simulink model "simulink2_dynamic_circle1"  (R2022a)
settings: Solver=FixedStepDiscrete  StartTime=0.0  StopTime=10.0  FixedStep=0.1  RelTol=1e-3
model workspace (MAT data in the model file):
  acceleration = 1
  alignment = 1
  cohesion = 1
  d_min = 0.5
  dt = 1
  eta = 1.5
  forward = 1
  k_ = 0.5
  k_tsmc = 1
  lambda_ = 2
  leader_position = [0 0 5]
  leader_velocity = [1 1 0]
  max_velocity = 5
  n_drones = 10
  neighbor_rad = 15
  radius = 10
  radius1 = 20
  ref_position = [20 20 5]
  ref_velocity = [0 0 0]
  separation = 1.5
  time_steps = 50
  u_max = 10
  velocities = [5 5 5]
  velocity = 5
settings Model: Creator=admin  LastModifiedBy=admin

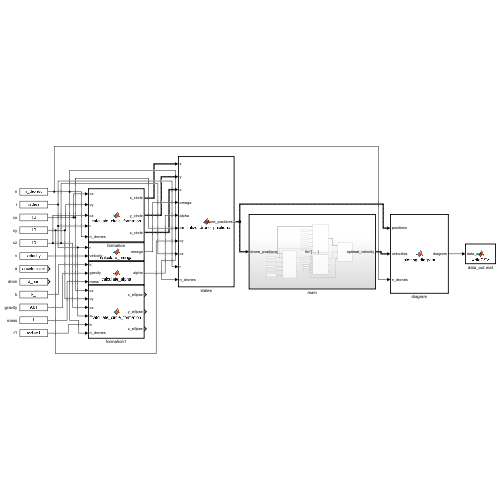
[thumbnail: Simulink's stored preview of the top-level diagram]
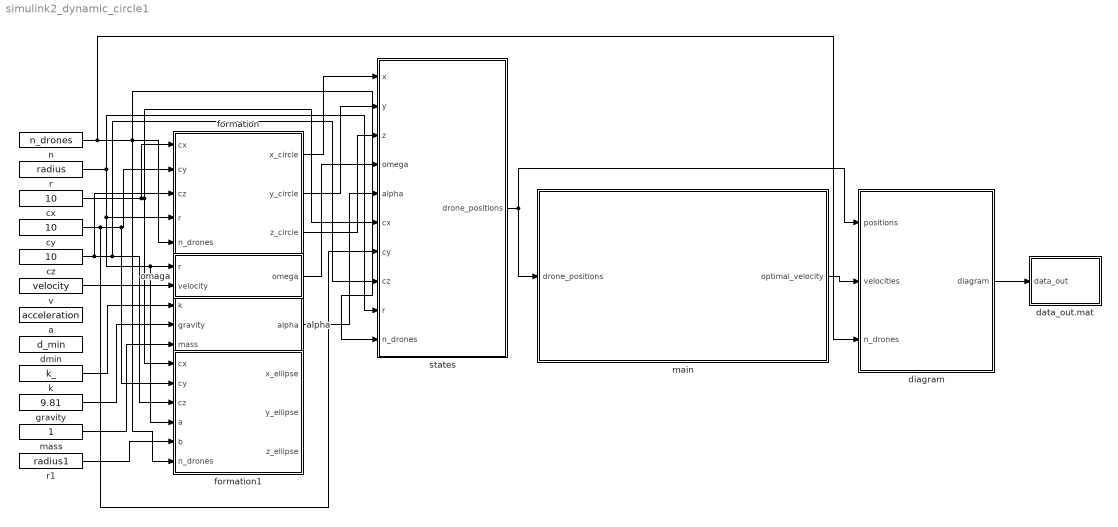
== system simulink2_dynamic_circle1 ==
  a : Constant  Value=acceleration
  alpha : MATLAB Function  TreatAsAtomicUnit=on
  cx : Constant  Value=10
  cy : Constant  Value=10
  cz : Constant  Value=10
  data_out.mat : MATLAB Function  TreatAsAtomicUnit=on
  diagram : MATLAB Function  TreatAsAtomicUnit=on
  dmin : Constant  Value=d_min
  formation : MATLAB Function  TreatAsAtomicUnit=on  SystemSampleTime=0.1
  formation1 : MATLAB Function  TreatAsAtomicUnit=on  SystemSampleTime=0.1
  gravity : Constant  Value=9.81
  k : Constant  Value=k_
  main : Subsystem  TreatAsAtomicUnit=on
  mass : Constant
  n : Constant  Value=n_drones
  omaga : MATLAB Function  TreatAsAtomicUnit=on
  r : Constant  Value=radius
  r1 : Constant  Value=radius1
  states : MATLAB Function  TreatAsAtomicUnit=on  SystemSampleTime=0.1
  v : Constant  Value=velocity
  wires:
  v/1 -> omaga/2(velocity)
  r/1 -> formation1/4(a), omaga/1(r), formation/4(r), states/9(r)
  k/1 -> alpha/1(k)
  gravity/1 -> alpha/2(gravity)
  mass/1 -> alpha/3(mass)
  cx/1 -> states/6(cx), formation1/1(cx), formation/1(cx)
  cy/1 -> states/7(cy), formation1/2(cy), formation/2(cy)
  cz/1 -> states/8(cz), formation1/3(cz), formation/3(cz)
  n/1 -> diagram/3(n_drones), states/10(n_drones), formation1/6(n_drones), formation/5(n_drones)
  r1/1 -> formation1/5(b)
  states/1(drone_positions) -> diagram/1(positions), main/1(drone_positions)
  formation/1(x_circle) -> states/1(x)
  formation/2(y_circle) -> states/2(y)
  formation/3(z_circle) -> states/3(z)
  omaga/1(omega) -> states/4(omega)
  alpha/1(alpha) -> states/5(alpha)
  main/1(optimal_velocity) -> diagram/2(velocities)
  diagram/1(diagram) -> data_out.mat/1(data_out)

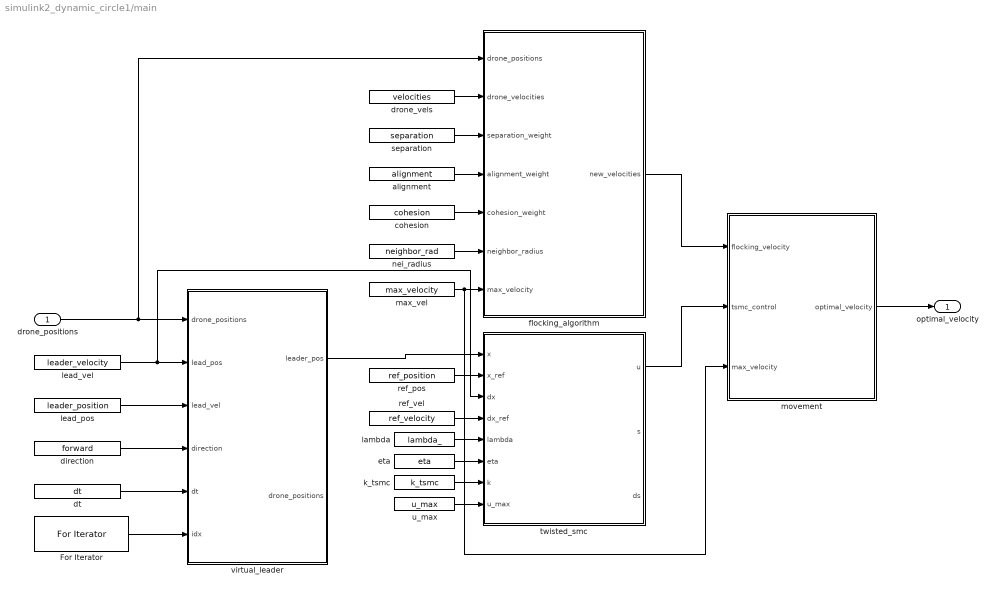
== system simulink2_dynamic_circle1/main ==
  drone_positions : Inport
  For Iterator : ForIterator  IterationLimit=time_steps
  alignment : Constant  Value=alignment
  cohesion : Constant  Value=cohesion
  direction : Constant  Value=forward
  drone_vels : Constant  Value=velocities
  dt : Constant  Value=dt
  eta : Constant  Value=eta
  flocking_algorithm : MATLAB Function  TreatAsAtomicUnit=on
  k_tsmc : Constant  Value=k_tsmc
  lambda : Constant  Value=lambda_
  lead_pos : Constant  Value=leader_position
  lead_vel : Constant  Value=leader_velocity
  max_vel : Constant  Value=max_velocity
  movement : MATLAB Function  TreatAsAtomicUnit=on
  nei_radius : Constant  Value=neighbor_rad
  ref_pos : Constant  Value=ref_position
  ref_vel : Constant  Value=ref_velocity
  separation : Constant  Value=separation
  twisted_smc : MATLAB Function  TreatAsAtomicUnit=on
  u_max : Constant  Value=u_max
  virtual_leader : MATLAB Function  TreatAsAtomicUnit=on
  optimal_velocity : Outport
  wires:
  dt/1 -> virtual_leader/5(dt)
  lead_vel/1 -> twisted_smc/3(dx), virtual_leader/2(lead_pos)
  direction/1 -> virtual_leader/4(direction)
  lead_pos/1 -> virtual_leader/3(lead_vel)
  drone_positions/1 -> flocking_algorithm/1(drone_positions), virtual_leader/1("drone_positions ")
  For Iterator/1 -> virtual_leader/6(idx)
  ref_vel/1 -> twisted_smc/4(dx_ref)
  ref_pos/1 -> twisted_smc/2(x_ref)
  virtual_leader/1(leader_pos) -> twisted_smc/1(x)
  lambda/1 -> twisted_smc/5(lambda)
  eta/1 -> twisted_smc/6(eta)
  k_tsmc/1 -> twisted_smc/7(k)
  u_max/1 -> twisted_smc/8(u_max)
  separation/1 -> flocking_algorithm/3(separation_weight)
  alignment/1 -> flocking_algorithm/4(alignment_weight)
  cohesion/1 -> flocking_algorithm/5(cohesion_weight)
  nei_radius/1 -> flocking_algorithm/6(neighbor_radius)
  max_vel/1 -> movement/3(max_velocity), flocking_algorithm/7(max_velocity)
  twisted_smc/1(u) -> movement/2(tsmc_control)
  flocking_algorithm/1(new_velocities) -> movement/1(flocking_velocity)
  drone_vels/1 -> flocking_algorithm/2(drone_velocities)
  movement/1(optimal_velocity) -> optimal_velocity/1

== matlab function simulink2_dynamic_circle1/main/virtual_leader ==
  data: drone_positions input; lead_pos input; leader_pos output; lead_vel input; direction input; dt input; drone_positions output; idx input
function [leader_pos, drone_positions] = virtual_leader(drone_positions, lead_pos, lead_vel, direction, dt, idx)
    switch direction
        case 1 % Forward
            lead_pos(1) = lead_pos(1) + lead_vel(1) * dt;
        case 2 % Backward
            lead_pos(1) = lead_pos(1) - lead_vel(1) * dt;
        case 3 % Left
            lead_pos(2) = lead_pos(2) - lead_vel(2) * dt;
        case 4 % Right
            lead_pos(2) = lead_pos(2) + lead_vel(2) * dt;
        case 5 % Up
            lead_pos(3) = lead_pos(3) + lead_vel(3) * dt;
        case 6 % Down
            lead_pos(3) = lead_pos(3) - lead_vel(3) * dt;
        otherwise
    end
    
    leader_pos = lead_pos;
end

== matlab function simulink2_dynamic_circle1/main/twisted_smc ==
  data: x input; u output; x_ref input; dx input; dx_ref input; lambda input; eta input; k input; u_max input; s output; ds output
function [u, s, ds] = twisted_sliding_control(x, x_ref, dx, dx_ref, lambda, eta, k, u_max)
    s = (x - x_ref) + lambda * (dx - dx_ref);
    ds = (dx - dx_ref) + lambda * (x - x_ref);

    u_eq = -lambda * dx;
    u_tsmc = k * sign(ds) - eta * sign(s);
    u = u_eq + u_tsmc;
    u = min(max(u, -u_max), u_max);
end

== matlab function simulink2_dynamic_circle1/main/flocking_algorithm ==
  data: drone_positions input; new_velocities output size=[1, 3]; drone_velocities input size=[1, 3]; separation_weight input; alignment_weight input; cohesion_weight input; neighbor_radius input; max_velocity input
function new_velocities = flocking_control_alpha_lattice(drone_positions, drone_velocities, separation_weight, alignment_weight, cohesion_weight, neighbor_radius, max_velocity)
    n_drones = size(drone_positions, 1);
    new_velocities = zeros(1, 3);
    
    for i = 1:n_drones
        current_position = drone_positions(i, :);

        separation_force = [0, 0, 0];
        alignment_force = [0, 0, 0];
        cohesion_force = [0, 0, 0];
        num_neighbors = 0;
        for j = 1:n_drones
            if i ~= j
                distance = norm(drone_positions(j, :) - current_position);
                if distance < neighbor_radius
                    separation_force = separation_force + (current_position - drone_positions(j, :)) / (distance^2);
                    alignment_force = alignment_force;
                    cohesion_force = cohesion_force + drone_positions(j, :);
                    num_neighbors = num_neighbors + 1;
                end
            end
        end

        if num_neighbors > 0
            alignment_force = (alignment_force / num_neighbors);
            alignment_force = alignment_weight * alignment_force;

            cohesion_force = (cohesion_force / num_neighbors) - current_position;
            cohesion_force = cohesion_weight * cohesion_force;

            separation_force = separation_weight * separation_force;
        end

        new_velocity = separation_force + alignment_force + cohesion_force;

        speed = norm(new_velocity);
        if speed > max_velocity
            new_velocity = (new_velocity / speed) * max_velocity;
        end

        new_velocities(1, :) = new_velocity;
    end
end

== matlab function simulink2_dynamic_circle1/main/movement ==
  data: flocking_velocity input size=[1, 3]; optimal_velocity output size=[n_drones, 3]; tsmc_control input; max_velocity input
function optimal_velocity = drone_movement(flocking_velocity, tsmc_control, max_velocity)
    tsmc_control = tsmc_control * ones(size(flocking_velocity));
    
    optimal_velocity = flocking_velocity + tsmc_control;

    speed = norm(optimal_velocity);
    if speed > max_velocity
        optimal_velocity = (optimal_velocity / speed) * max_velocity;
    end
end

== matlab function simulink2_dynamic_circle1/diagram ==
  data: positions input; velocities input; n_drones input; diagram output size=[15000, 12]
function diagram = plotting_diagram(positions, velocities, n_drones)
    figure_handle1 = figure;
    figure_handle2 = figure;
    r = 10;
    cx = 0;
    cy = 0;
    cz = 5;
    
    dt = 1;
    total_time = 50;
    time_steps = total_time / dt;
    full_data_record = [];
    for t = 1:time_steps
        % Plot formation
        data_out = plot_formation(positions, r, cx, cy, cz, t, dt, figure_handle1, figure_handle2);
        full_data_record = [full_data_record; data_out]; %#ok<AGROW>
        pause(0.1);
    end
    diagram = full_data_record; 
end

function data_out = plot_formation(~, r, cx, cy, cz, t, dt, figure_handle1, figure_handle2)
    persistent previous_formation data_record data_record_counter time_series_data trail_data;
    
    if isempty(previous_formation)
        n_drones = 10;
        previous_formation = [cx + rand(1, n_drones)' * r, cy + rand(1, n_drones)' * r, cz * ones(n_drones, 1)];
        active_drones = n_drones;
        data_record = zeros(1000, 12);
        data_record_counter = 0;
        time_series_data.time = zeros(1, 1000);
        time_series_data.z = zeros(1000, n_drones);
        time_series_data.roll = zeros(1000, n_drones);
        time_series_data.pitch = zeros(1000, n_drones);
        time_series_data.yaw = zeros(1000, n_drones);
        trail_data.x = cell(1, n_drones);
        trail_data.y = cell(1, n_drones);
        trail_data.z = cell(1, n_drones);
        for i = 1:n_drones
            trail_data.x{i} = nan(1, 1000);
            trail_data.y{i} = nan(1, 1000);
            trail_data.z{i} = nan(1, 1000);
        end
    end

    active_drones = size(previous_formation, 1);

    if t <= 20
        active_drones = 10;
    elseif t > 20 && t <= 30
        active_drones = max(4, active_drones - 1);
    elseif t > 30 && t <= 40
        active_drones = min(10, active_drones + 1);
    end
    
    n_drones = size(previous_formation, 1);
    centroid = mean(previous_formation, 1);
    

%     x_target = centroid(1) + (r * 1.5) * cos((2 * pi * (0:n_drones-1)) / n_drones);
%     y_target = centroid(2) + r * sin((2 * pi * (0:n_drones-1)) / n_drones);
%     z_target = centroid(3) * ones(1, n_drones);
%     outer_shape = 'ellipse';

    x_target = centroid(1) + r * cos((2 * pi * (0:n_drones-1)) / n_drones);
    y_target = centroid(2) + r * sin((2 * pi * (0:n_drones-1)) / n_drones);
    z_target = centroid(3) * ones(1, n_drones);
    outer_shape = 'circle';

%     x_target = linspace(centroid(1) - r, centroid(1) + r, n_drones);
%     y_target = centroid(2) * ones(1, n_drones);
%     z_target = centroid(3) * ones(1, n_drones);
%     outer_shape = 'line';

%     x_target = centroid(1) + (r * 1.5) * cos((2 * pi * (0:n_drones-1)) / n_drones);
%     y_target = centroid(2) + r * sin((2 * pi * (0:n_drones-1)) / n_drones);
%     z_target = centroid(3) * ones(1, n_drones);
%     outer_shape = 'ellipse';

    if t > 1 && t <= 10
        x_target = x_target + 5;
    elseif t > 10 && t <= 20
        y_target = y_target + 5;
    elseif t > 20 && t <= 30
        x_target = x_target - 5;
    elseif t > 30 && t <= 40
        y_target = y_target - 5;
    elseif t > 40
        angle_increment = 2 * pi * ((t - 20) / 30);
        z_increment = min(4 * ((t - 20) / 30), 4);
        
        rotation_matrix = [cos(angle_increment), -sin(angle_increment), 0;
                           sin(angle_increment),  cos(angle_increment), 0;
                           0,                     0,                    1];
        
        rotated_positions = rotation_matrix * [x_target - centroid(1); y_target - centroid(2); z_target - centroid(3)];
        x_target = rotated_positions(1, :) + centroid(1);
        y_target = rotated_positions(2, :) + centroid(2);
        z_target = rotated_positions(3, :) + centroid(3) + z_increment;
    end

    for i = 1:n_drones
        if i > active_drones
            x_target(i) = x_target(i) + 10 * sign(x_target(i) - centroid(1));
            y_target(i) = y_target(i) + 10 * sign(y_target(i) - centroid(2));
        end
    end

    smoothing_factor = 0.5;
    x_formation = previous_formation(:, 1)' + (x_target - previous_formation(:, 1)') * smoothing_factor;
    y_formation = previous_formation(:, 2)' + (y_target - previous_formation(:, 2)') * smoothing_factor;
    z_formation = previous_formation(:, 3)' + (z_target - previous_formation(:, 3)') * smoothing_factor;
    roll_actual = rand(1, n_drones) * 5;
    pitch_actual = rand(1, n_drones) * 5;
    yaw_actual = rand(1, n_drones) * 5;
    
    % Simulasi data motor
    motor_speed_x = rand(1, n_drones) * 100; % Kecepatan motor pada sumbu X (unit disesuaikan)
    motor_speed_y = rand(1, n_drones) * 100; % Kecepatan motor pada sumbu Y
    motor_speed_z = rand(1, n_drones) * 100; % Kecepatan motor pada sumbu Z
    
    % Hitung RMSE
    error_x = sqrt(mean((x_target - x_formation).^2));
    error_y = sqrt(mean((y_target - y_formation).^2));
    error_z = sqrt(mean((z_target - z_formation).^2));
    rmse = sqrt((error_x^2 + error_y^2 + error_z^2) / 3);
    for i = 1:n_drones
        data_record_counter = data_record_counter + 1;
        data_record(data_record_counter, :) = [t, i, x_formation(i), y_formation(i), z_formation(i), ...
                                               roll_actual(i), pitch_actual(i), yaw_actual(i), ...
                                               motor_speed_x(i), motor_speed_y(i), motor_speed_z(i), rmse];
        if data_record_counter <= length(trail_data.x{i})
            trail_data.x{i}(data_record_counter) = x_formation(i);
            trail_data.y{i}(data_record_counter) = y_formation(i);
            trail_data.z{i}(data_record_counter) = z_formation(i);
        end
    end
    
    time_series_data.time(t) = t;
    time_series_data.z(t, :) = z_formation;
    time_series_data.roll(t, :) = roll_actual;
    time_series_data.pitch(t, :) = pitch_actual;
    time_series_data.yaw(t, :) = yaw_actual;

    previous_formation = [x_formation', y_formation', z_formation'];

    figure(figure_handle1);
    clf;

    plot3(x_formation(1:active_drones), y_formation(1:active_drones), z_formation(1:active_drones), 'ro', 'MarkerSize', 5);
    hold on;
    
    for i = 1:active_drones
        text(x_formation(i), y_formation(i), z_formation(i), sprintf('%d', int32(i)), 'VerticalAlignment', 'bottom', 'HorizontalAlignment', 'right');
    end

    for i = 1:n_drones
        plot3(trail_data.x{i}(~isnan(trail_data.x{i})), trail_data.y{i}(~isnan(trail_data.y{i})), ...
              trail_data.z{i}(~isnan(trail_data.z{i})), 'Color', [0.5 0.5 0.5], 'LineStyle', '--');
    end

    for i = 1:active_drones
        next_index = mod(i, active_drones) + 1;
        plot3([x_formation(i), x_formation(next_index)], ...
              [y_formation(i), y_formation(next_index)], ...
              [z_formation(i), z_formation(next_index)], ...
              'r-');
    end
   
    theta = linspace(0, 2 * pi, 100);
    x_outer = zeros(1, 100);
    y_outer = zeros(1, 100);
    z_outer = zeros(1, 100);

    switch outer_shape
        case 'line'
            x_outer = linspace(centroid(1) - r, centroid(1) + r, 100);
            y_outer = centroid(2) * ones(1, 100);
            z_outer = centroid(3) * ones(1, 100);
        case 'circle'
            x_outer = centroid(1) + r * cos(theta);
            y_outer = centroid(2) + r * sin(theta);
            z_outer = centroid(3) * ones(1, length(theta));
        case 'ellipse'
            x_outer = centroid(1) + (r * 1.5) * cos(theta);
            y_outer = centroid(2) + r * sin(theta);
            z_outer = centroid(3) * ones(1, length(theta));
    end
    
    plot3(x_outer, y_outer, z_outer, 'k--', 'LineWidth', 1);

%     if t <= 16
%         text(x_formation(1), y_formation(1), z_formation(1), 'Line Formation', 'Color', 'red');
%     elseif t <= 33
%         text(x_formation(1), y_formation(1), z_formation(1), 'Circle Formation', 'Color', 'red');
%     elseif t <= 49
%         text(x_formation(1), y_formation(1), z_formation(1), 'Ellipsis Formation', 'Color', 'red');
%     else
%         text(x_formation(1), y_formation(1), z_formation(1), 'Spiral Formation', 'Color', 'red');
%     end
    
    xlabel('X');
    ylabel('Y');
    zlabel('Z');
    title(['Time: ', sprintf('%0.2f', t * dt)]);
    axis equal;
    grid on;
    axis([-50 50 -50 50 0 50]);
    drawnow;



    figure(figure_handle2);

    subplot(4, 1, 1);
    plot(time_series_data.time, time_series_data.z);
    title('Z Position of Drones Over Time');
    xlabel('Time');
    ylabel('Z Position');
    ylim([0, 20]);
    subplot(4, 1, 2);
    plot(time_series_data.time, time_series_data.roll);
    title('Roll of Drones Over Time');
    xlabel('Time');
    ylabel('Roll (degrees)');
    ylim([0, 20]);
    subplot(4, 1, 3);
    plot(time_series_data.time, time_series_data.pitch);
    title('Pitch of Drones Over Time');
    xlabel('Time');
    ylabel('Pitch (degrees)');
    ylim([0, 20]);
    subplot(4, 1, 4);
    plot(time_series_data.time, time_series_data.yaw);
    title('Yaw of Drones Over Time');
    xlabel('Time');
    ylabel('Yaw (degrees)');
    ylim([0, 20]);

    drawnow;

    data_out = data_record(1:data_record_counter, :);
end

== matlab function simulink2_dynamic_circle1/data_out.mat ==
  data: data_out input
function writeCSV(data_out)
    coder.extrinsic('writematrix');
    coder.extrinsic('fileID', 'fprintf', 'fclose'); 
    headers = {'Time (s)', 'Drone ID', 'X Position (m)', 'Y Position (m)', 'Z Position (m)', ...
               'Roll (deg)', 'Pitch (deg)', 'Yaw (deg)', 'Motor Speed X (RPM)', 'Motor Speed Y (RPM)', 'Motor Speed Z (RPM)', ...
               'RMSE (m)', 'X Position Actual (m)', 'Y Position Actual (m)', 'Z Position Actual (m)'};

    x_actual = data_out(:, 3) + (data_out(:, 12) / 20);
    y_actual = data_out(:, 4) + (data_out(:, 12) / 20);
    z_actual = data_out(:, 5) + (data_out(:, 12) / 20);
    data_out(:, 12) = (data_out(:, 12) / 20);
    data_out = [data_out, x_actual, y_actual, z_actual];

    fileID = fopen('dynamic_drone_data_file6.csv', 'w');
    fprintf(fileID, '%s,', headers{1:end-1});
    fprintf(fileID, '%s\n', headers{end});
    fclose(fileID);

    writematrix(data_out, 'dynamic_drone_data_file6.csv', 'WriteMode', 'append');
end

== matlab function simulink2_dynamic_circle1/alpha ==
  data: k input; alpha output; gravity input; mass input
function alpha = calculate_alpha(k, gravity, mass)
    alpha = k * (gravity / mass);
end

== matlab function simulink2_dynamic_circle1/omaga ==
  data: r input; velocity input; omega output
function omega = calculate_omega(r, velocity)
    omega = (2 * pi * velocity) / r;
end

== matlab function simulink2_dynamic_circle1/formation ==
  data: cx input; x_circle output size=[1, n_drones]; cy input; cz input; r input; n_drones input; y_circle output size=[1, n_drones]; z_circle output size=[1, n_drones]
function [x_circle, y_circle, z_circle] = calculate_circle_formation(cx, cy, cz, r, n_drones)
    theta = (2 * pi * (0:n_drones-1)) / n_drones;
    
    x_circle = cx + r * cos(theta);
    y_circle = cy + r * sin(theta);
    z_circle = cz * ones(1, n_drones);
end

== matlab function simulink2_dynamic_circle1/formation1 ==
  data: cx input; x_ellipse output size=[1, n_drones]; cy input; cz input; a input; b input; n_drones input; y_ellipse output size=[1, n_drones]; z_ellipse output size=[1, n_drones]
function [x_ellipse, y_ellipse, z_ellipse] = calculate_circle_formation(cx, cy, cz, a, b, n_drones)
    
    x_ellipse = cx + a * cos((2 * pi * (0:n_drones-1)) / n_drones);
    y_ellipse = cy + b * sin((2 * pi * (0:n_drones-1)) / n_drones);
    z_ellipse = cz * ones(1, n_drones);

end

== matlab function simulink2_dynamic_circle1/states ==
  data: x input; y input; z input; omega input; alpha input; cx input; drone_positions output size=[n_drones, 3]; cy input; cz input; r input; n_drones input
function drone_positions = initialize_drone_positions(x, y, z, omega, alpha, cx, cy, cz, r, n_drones)
    theta = (2 * pi * (0:n_drones-1)) / n_drones;
    
    x_positions = cx + r * cos(theta); % 1 x n_drones
    y_positions = cy + r * sin(theta); % 1 x n_drones
    z_positions = cz * ones(1, n_drones); % 1 x n_drones
    
    drone_positions = [x_positions; y_positions; z_positions]';
end
